simulink model "controler"  (Simulink 8.3)
settings: Solver=FixedStepDiscrete  StartTime=0.0  StopTime=10.0  RelTol=1e-3
values from neighbouring files (symbols this model uses):
  ki_teta = omega*omega/alpha    (= 0.2)    [InitRobotAndEnvironment.m]    (also in sampling.m)
  kp_teta = 2*ksi*omega/alpha    (= 0.4)    [InitRobotAndEnvironment.m]    (also in sampling.m)
libraries: simulink x2
settings Model: Creator=gallets  LastModifiedBy=gallets
settings DataIOCC: SignalLoggingSaveFormat=Dataset
settings DebuggingCC: AlgebraicLoopMsg=error  UnderspecifiedInitializationDetection=Simplified  StateNameClashWarn=none
settings GRTTargetCC: CombineOutputUpdateFcns=on  GRTInterface=off

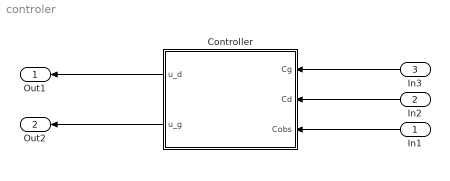
== system controler ==
  In1 : Inport
  In2 : Inport  Port=2
  In3 : Inport  Port=3
  Controller : Subsystem
  Out1 : Outport
  Out2 : Outport  Port=2
  wires:
  In2/1 -> Controller/2(Cd)
  In3/1 -> Controller/1(Cg)
  In1/1 -> Controller/3("Cobs ")
  Controller/1(u_d) -> Out1/1
  Controller/2(u_g) -> Out2/1

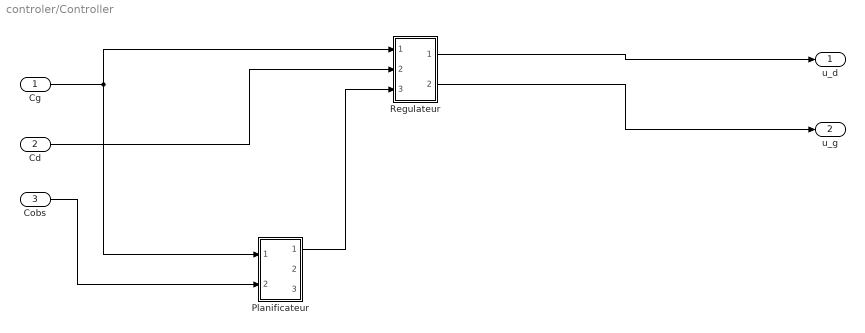
== system controler/Controller ==
  Cg : Inport
  Cd : Inport  Port=2
  "Cobs " : Inport  Port=3
  Planificateur : Subsystem
  Regulateur : Subsystem
  u_d : Outport
  u_g : Outport  Port=2
  wires:
  Cg/1 -> Planificateur/1(In1), Regulateur/1(In1)
  Cd/1 -> Regulateur/2(In2)
  Regulateur/1(Out1) -> u_d/1
  Regulateur/2(Out2) -> u_g/1
  "Cobs "/1 -> Planificateur/2(In2)
  Planificateur/1(Out1) -> Regulateur/3(In3)

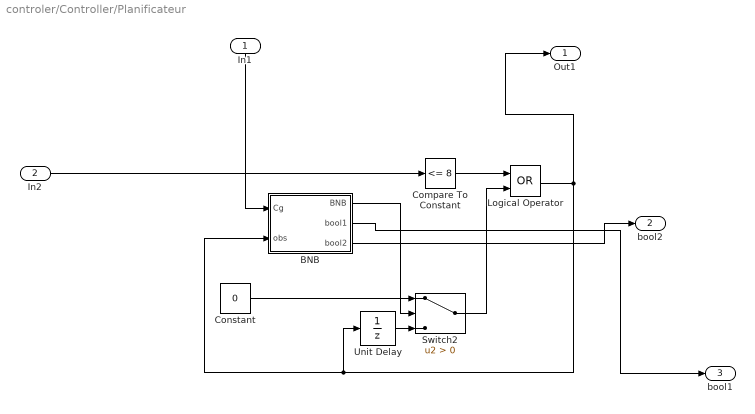
== system controler/Controller/Planificateur ==
  In1 : Inport  OutDataTypeStr=double
  In2 : Inport  Port=2  OutDataTypeStr=double
  BNB : Subsystem
  Compare To Constant : simulink/Logic and Bit Operations/Compare To Constant  relop=<=  const=8  OutDataTypeStr=boolean
  Constant : Constant  Value=0
  Logical Operator : Logic  Operator=OR  AllPortsSameDT=off  OutDataTypeStr=boolean
  Switch2 : Switch  Criteria=u2 > Threshold
  Unit Delay : UnitDelay  SampleTime=-1
  Out1 : Outport
  bool2 : Outport  Port=2
  bool1 : Outport  Port=3
  wires:
  In1/1 -> BNB/1(Cg)
  BNB/1("BNB ") -> Switch2/2
  Compare To Constant/1 -> Logical Operator/1
  Logical Operator/1 -> BNB/2(obs), Unit Delay/1, Out1/1
  Switch2/1 -> Logical Operator/2
  Constant/1 -> Switch2/1
  In2/1 -> Compare To Constant/1
  Unit Delay/1 -> Switch2/3
  BNB/3(bool2) -> bool2/1
  BNB/2(bool1) -> bool1/1

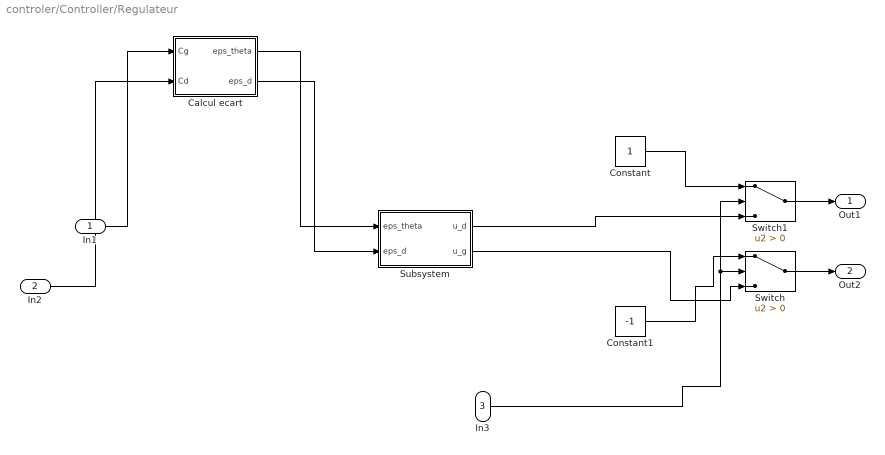
== system controler/Controller/Regulateur ==
  In1 : Inport
  In2 : Inport  Port=2
  In3 : Inport  Port=3  OutDataTypeStr=double
  Calcul ecart : Subsystem
  Constant : Constant
  Constant1 : Constant  Value=-1
  Subsystem : Subsystem
  Switch : Switch  Criteria=u2 > Threshold
  Switch1 : Switch  Criteria=u2 > Threshold
  Out1 : Outport
  Out2 : Outport  Port=2
  wires:
  In3/1 -> Switch1/2, Switch/2
  In1/1 -> Calcul ecart/1(Cg)
  Subsystem/2(u_g) -> Switch/3
  Subsystem/1(u_d) -> Switch1/3
  Calcul ecart/2(eps_d) -> Subsystem/2(eps_d)
  In2/1 -> Calcul ecart/2(Cd)
  Calcul ecart/1(eps_theta) -> Subsystem/1(eps_theta)
  Switch/1 -> Out2/1
  Switch1/1 -> Out1/1
  Constant/1 -> Switch1/1
  Constant1/1 -> Switch/1

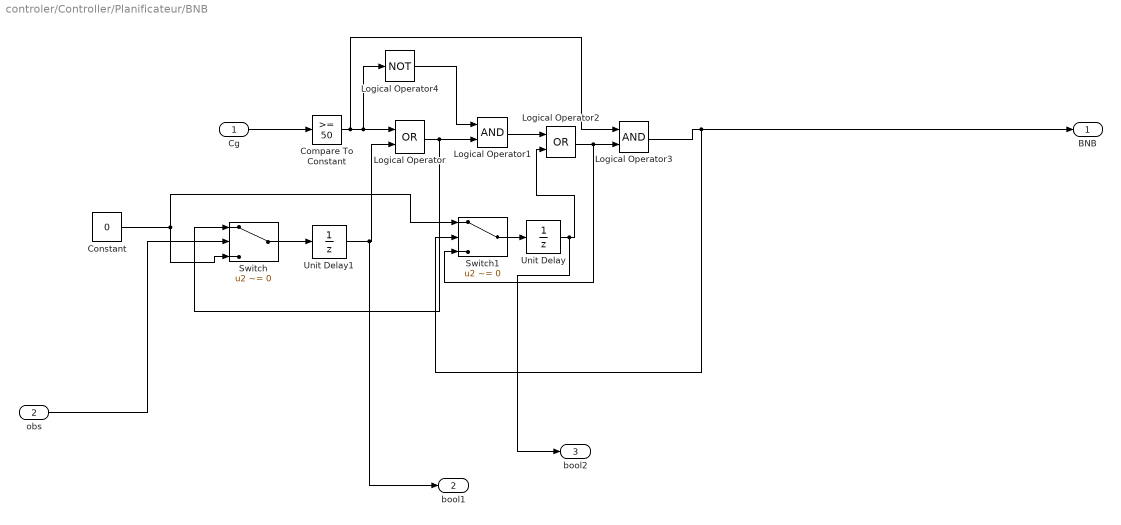
== system controler/Controller/Planificateur/BNB ==
  Cg : Inport
  obs : Inport  Port=2
  Compare To Constant : simulink/Logic and Bit Operations/Compare To Constant  relop=>=  const=50  OutDataTypeStr=boolean
  Constant : Constant  Value=0
  Logical Operator : Logic  Operator=OR  AllPortsSameDT=off  OutDataTypeStr=boolean
  Logical Operator1 : Logic  AllPortsSameDT=off  OutDataTypeStr=boolean
  Logical Operator2 : Logic  Operator=OR  AllPortsSameDT=off  OutDataTypeStr=boolean
  Logical Operator3 : Logic  AllPortsSameDT=off  OutDataTypeStr=boolean
  Logical Operator4 : Logic  Operator=NOT  AllPortsSameDT=off  OutDataTypeStr=boolean
  Switch : Switch  Criteria=u2 ~= 0
  Switch1 : Switch  Criteria=u2 ~= 0
  Unit Delay : UnitDelay  SampleTime=-1
  Unit Delay1 : UnitDelay  SampleTime=-1
  "BNB " : Outport
  bool1 : Outport  Port=2
  bool2 : Outport  Port=3
  wires:
  Logical Operator/1 -> Switch/1, Logical Operator1/2
  Unit Delay1/1 -> bool1/1, Logical Operator/2
  Compare To Constant/1 -> Logical Operator3/1, Logical Operator4/1, Logical Operator/1
  Logical Operator1/1 -> Logical Operator2/1
  Logical Operator2/1 -> Switch1/3, Logical Operator3/2
  Unit Delay/1 -> bool2/1, Logical Operator2/2
  Constant/1 -> Switch/3, Switch1/1
  Switch/1 -> Unit Delay1/1
  Switch1/1 -> Unit Delay/1
  Logical Operator4/1 -> Logical Operator1/1
  Cg/1 -> Compare To Constant/1
  Logical Operator3/1 -> "BNB "/1, Switch1/2
  obs/1 -> Switch/2

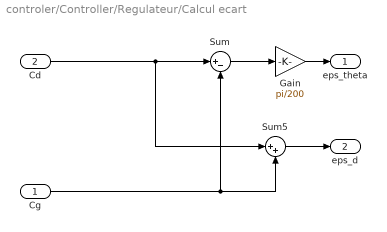
== system controler/Controller/Regulateur/Calcul ecart ==
  Cg : Inport
  Cd : Inport  Port=2
  Gain : Gain  Gain=pi/200
  Sum : Sum  Inputs=|+-
  Sum5 : Sum  Inputs=|++
  eps_theta : Outport
  eps_d : Outport  Port=2
  wires:
  Sum/1 -> Gain/1
  Cd/1 -> Sum/1, Sum5/1
  Cg/1 -> Sum/2, Sum5/2
  Gain/1 -> eps_theta/1
  Sum5/1 -> eps_d/1

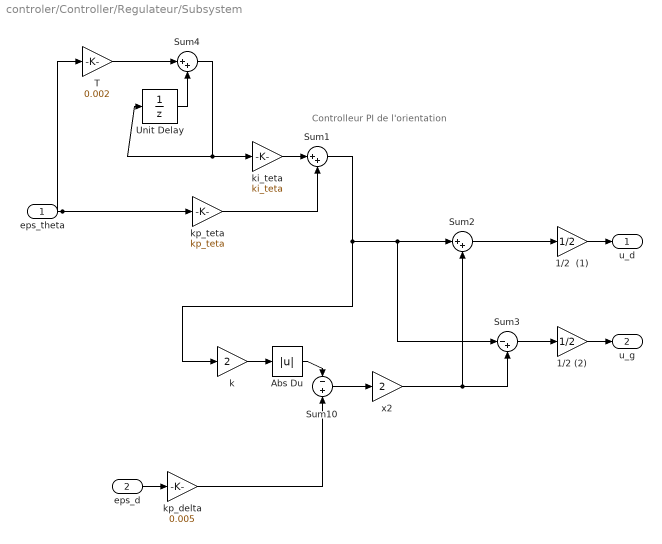
== system controler/Controller/Regulateur/Subsystem ==
  note: Controlleur PI de l'orientation
  eps_theta : Inport
  eps_d : Inport  Port=2
  1/2  (1) : Gain  Gain=1/2  SaturateOnIntegerOverflow=on  OutDataTypeStr=Inherit: Same as input  ParamDataTypeStr=Inherit: Same as input
  1/2 (2) : Gain  Gain=1/2  SaturateOnIntegerOverflow=on  OutDataTypeStr=Inherit: Same as input  ParamDataTypeStr=Inherit: Same as input
  Abs Du : Abs  SaturateOnIntegerOverflow=on
  Sum1 : Sum  Inputs=|++  SaturateOnIntegerOverflow=on
  Sum10 : Sum  Inputs=-+  SaturateOnIntegerOverflow=on
  Sum2 : Sum  Inputs=|++  SaturateOnIntegerOverflow=on
  Sum3 : Sum  Inputs=|-+  SaturateOnIntegerOverflow=on
  Sum4 : Sum  Inputs=|++
  T : Gain  Gain=0.002
  Unit Delay : UnitDelay  SampleTime=-1
  k : Gain  Gain=2  SaturateOnIntegerOverflow=on  OutDataTypeStr=Inherit: Same as input  ParamDataTypeStr=Inherit: Same as input
  ki_teta : Gain  Gain=ki_teta  SaturateOnIntegerOverflow=on  OutDataTypeStr=Inherit: Same as input  ParamDataTypeStr=Inherit: Same as input
  kp_delta : Gain  Gain=0.005
  kp_teta : Gain  Gain=kp_teta  SaturateOnIntegerOverflow=on  OutDataTypeStr=Inherit: Same as input  ParamDataTypeStr=Inherit: Same as input
  x2 : Gain  Gain=2  SaturateOnIntegerOverflow=on  OutDataTypeStr=Inherit: Same as input  ParamDataTypeStr=Inherit: Same as input
  u_d : Outport
  u_g : Outport  Port=2
  wires:
  ki_teta/1 -> Sum1/1
  kp_teta/1 -> Sum1/2
  Sum2/1 -> 1/2  (1)/1
  Sum3/1 -> 1/2 (2)/1
  k/1 -> Abs Du/1
  kp_delta/1 -> Sum10/2
  eps_theta/1 -> kp_teta/1, T/1
  Abs Du/1 -> Sum10/1
  x2/1 -> Sum2/2, Sum3/2
  Sum10/1 -> x2/1
  Sum1/1 -> k/1, Sum2/1, Sum3/1
  T/1 -> Sum4/1
  Sum4/1 -> ki_teta/1, Unit Delay/1
  Unit Delay/1 -> Sum4/2
  1/2  (1)/1 -> u_d/1
  1/2 (2)/1 -> u_g/1
  eps_d/1 -> kp_delta/1
